simulink subsystem "Trans_update"  (R2025b)
settings: Solver=VariableStepAuto  StartTime=0.0  StopTime=10.0  RelTol=1e-3
settings Model: Creator=Admin  LastModifiedBy=Admin

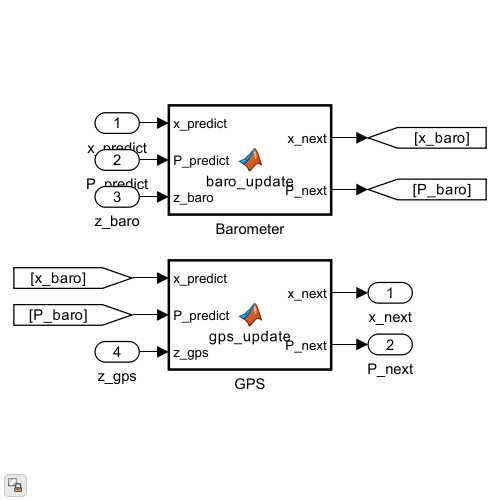
[thumbnail: Simulink's stored preview of the top-level diagram]
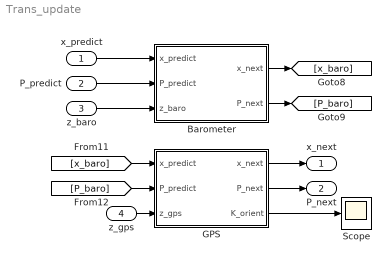
== system Trans_update ==
  x_predict : Inport
  P_predict : Inport  Port=2
  z_baro : Inport  Port=3
  z_gps : Inport  Port=4
  Barometer : MATLAB Function  TreatAsAtomicUnit=on
  GPS : MATLAB Function  TreatAsAtomicUnit=on
  Scope : Scope
      settings: ActiveDisplayYMinimum=-1  ActiveDisplayYMaximum=1
  x_next : Outport
  P_next : Outport  Port=2
  wires:
  Barometer/2(P_next) -> [P_baro]
  z_gps/1 -> GPS/3(z_gps)
  P_predict/1 -> Barometer/2(P_predict)
  Barometer/1(x_next) -> [x_baro]
  x_predict/1 -> Barometer/1(x_predict)
  z_baro/1 -> Barometer/3(z_baro)
  [x_baro] -> GPS/1(x_predict)
  [P_baro] -> GPS/2(P_predict)
  GPS/2(P_next) -> P_next/1
  GPS/1(x_next) -> x_next/1
  GPS/3(K_orient) -> Scope/1

== matlab function Trans_update/Barometer ==
  data: x_predict input; x_next output; P_predict input; z_baro input; P_next output
function [x_next, P_next] = baro_update(x_predict, P_predict, z_baro)

% x = [p(3); v(3); q(4); bg(3); ba_high(3); ba_low(3)]   -> 19 states

% Measurement noise
sigma_T = 0.05;       % K
sigma_P = 10;       % Pa
R = diag([sigma_T^2, sigma_P^2]);
n = 19;

% Constants
P_surface = 101325;
T_surface = 288.15;
M_0       = 28.9644e-3;   % kg/mol
R_gas     = 8.31446;      % J/(mol*K)
g_0       = 9.80665;
L         = -0.0065;      % K/m

% If state uses NED, x(3) is Down, so altitude is negative of that
h = -x_predict(3);

% Predicted measurements
T_pred = T_surface + L * h;
exponent = (g_0 * M_0) / (R_gas * L);
P_pred = P_surface * (T_surface / T_pred)^exponent;

% Derivatives w.r.t. altitude h
dT_dh = L;
dP_dh = -exponent * L * P_pred / T_pred;

% Jacobian w.r.t. state x
% since h = -x(3), dz/dx(3) = dz/dh * (-1)
H = zeros(2,n);
H(1,3) = -dT_dh;
H(2,3) = -dP_dh;

% Innovation
y = z_baro(:) - [T_pred; P_pred];

% Kalman update
S   = H * P_predict * H' + R;
K_k = P_predict * H' / S;
x_next = x_predict + K_k * y;

% Add before the Joseph covariance update
x_next(7:10) = x_next(7:10) / norm(x_next(7:10));

% Joseph form
IKH    = eye(n) - K_k * H;
P_next = IKH * P_predict * IKH' + K_k * R * K_k';

end

== matlab function Trans_update/GPS ==
  data: x_predict input; x_next output; P_predict input; z_gps input; P_next output; K_orient output
function [x_next, P_next, K_orient] = gps_update(x_predict, P_predict, z_gps)
% x = [p(3); v(3); q(4); bg(3); ba_high(3); ba_low(3)] -> 19 states
% z_gps = [lat; lon; h; vN; vE; vD; fix; sat; pdop]

% Reference origin
lat0_deg = 51.507351;
lon0_deg = -0.127758;
h0       = 25;
n = 19;
K_orient = zeros(4, 6);

% GPS quality gate
if z_gps(7) < 1 || z_gps(8) < 4 || z_gps(9) > 3.0
    x_next = x_predict;
    P_next = P_predict;
    return;
end

% Unpack
lat_deg = z_gps(1);
lon_deg = z_gps(2);
h_alt   = z_gps(3);
v_ned   = z_gps(4:6);

% WGS84 constants
a_earth = 6378137.0;
e2      = 0.00669437999014;

% Convert degrees to radians
lat0 = deg2rad(lat0_deg);
lon0 = deg2rad(lon0_deg);
lat  = deg2rad(lat_deg);
lon  = deg2rad(lon_deg);

% LLA -> ECEF (measurement)
N_curve = a_earth / sqrt(1 - e2 * sin(lat)^2);
X = (N_curve + h_alt) * cos(lat) * cos(lon);
Y = (N_curve + h_alt) * cos(lat) * sin(lon);
Z = (N_curve * (1 - e2) + h_alt) * sin(lat);

% LLA -> ECEF (reference)
N0 = a_earth / sqrt(1 - e2 * sin(lat0)^2);
X0 = (N0 + h0) * cos(lat0) * cos(lon0);
Y0 = (N0 + h0) * cos(lat0) * sin(lon0);
Z0 = (N0 * (1 - e2) + h0) * sin(lat0);

% ECEF delta -> NED
dX = X - X0;  dY = Y - Y0;  dZ = Z - Z0;

pN =  -sin(lat0)*cos(lon0)*dX - sin(lat0)*sin(lon0)*dY + cos(lat0)*dZ;
pE =  -sin(lon0)*dX            + cos(lon0)*dY;
pD =  -cos(lat0)*cos(lon0)*dX - cos(lat0)*sin(lon0)*dY - sin(lat0)*dZ;

% Position + velocity measurement
z      = [pN; pE; pD; v_ned(:)];
h_pred = [x_predict(1:3); x_predict(4:6)];

% Measurement noise
sigma_pos_h = 1;
sigma_pos_v = 2.5;
sigma_vel_h = 10;   % from corrected characterisation
sigma_vel_v = 10;
R = diag([sigma_pos_h^2, sigma_pos_h^2, sigma_pos_v^2, ...
          sigma_vel_h^2, sigma_vel_h^2, sigma_vel_v^2]);

% Jacobian (6 x 19)
H = zeros(6, n);
H(1:3, 1:3) = eye(3);   % position
H(4:6, 4:6) = eye(3);   % velocity

% Innovation
y = z - h_pred;

% Innovation gating (chi-squared, 6 DOF — threshold updated from 3 DOF)
S = H * P_predict * H' + R;

% Kalman gain and update
K      = P_predict * H' / S;
K_orient = K(7:10, :);
x_next = x_predict + K * y;
x_next(7:10) = x_next(7:10) / norm(x_next(7:10));

% Joseph form
IKH    = eye(n) - K * H;
P_next = IKH * P_predict * IKH' + K * R * K';
end
